simulink model "gaps_ut"  (Simulink 8.1)
settings: Solver=FixedStepDiscrete  StartTime=0.0  StopTime=10.0  FixedStep=0.005  RelTol=1e-3
libraries: siltestlib x11, gaps x1
settings Model: Creator=AT015126  LastModifiedBy=AT015555
settings DataIOCC: SignalLoggingSaveFormat=Dataset
settings OptimizationCC: ExpressionDepthLimit=128
settings DebuggingCC: FcnCallInpInsideContextMsg=EnableAllAsError
settings GRTTargetCC: CombineOutputUpdateFcns=on  GRTInterface=off

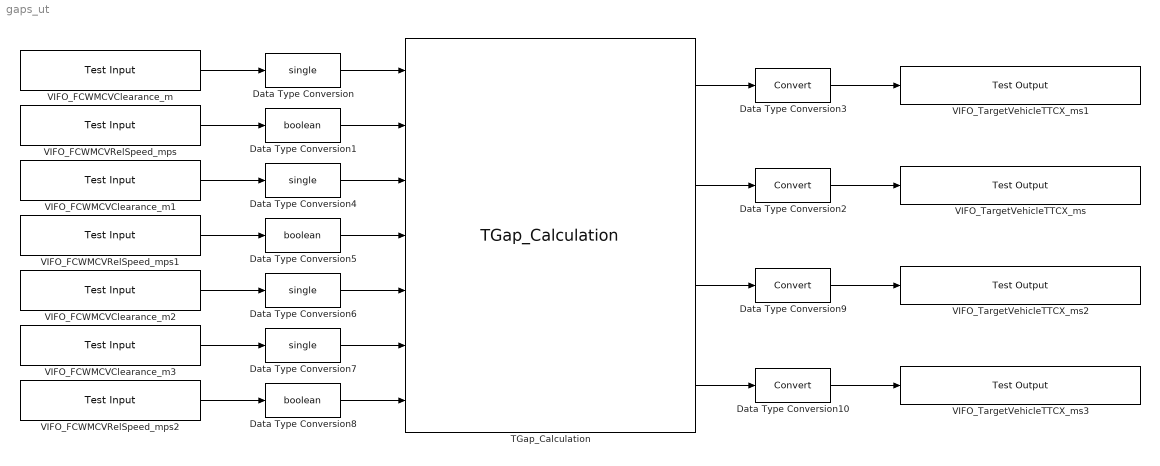
== system gaps_ut ==
  Data Type Conversion{,4,6..7} (4 alike) : DataTypeConversion  OutDataTypeStr=single
  Data Type Conversion1 : DataTypeConversion  OutDataTypeStr=boolean
  Data Type Conversion{2..3,9..10} (4 alike) : DataTypeConversion
  Data Type Conversion5 : DataTypeConversion  OutDataTypeStr=boolean
  Data Type Conversion8 : DataTypeConversion  OutDataTypeStr=boolean
  TGap_Calculation : gaps/TGap_Calculation
  VIFO_FCWMCVClearance_m : siltestlib/Test Input  varname=VIFO_AEBVehClearance_m  sampletime=0.005
  VIFO_FCWMCVClearance_m1 : siltestlib/Test Input  varname=VIFO_ACCMCVehXPosition_m  sampletime=0.005
  VIFO_FCWMCVClearance_m2 : siltestlib/Test Input  varname=VDINR_VehSpd_mps  sampletime=0.005
  VIFO_FCWMCVClearance_m3 : siltestlib/Test Input  varname=VIFO_FCWVehClearance_m  sampletime=0.005
  VIFO_FCWMCVRelSpeed_mps : siltestlib/Test Input  varname=VIFO_AEBTargetVehAssigned_flg  sampletime=0.005
  VIFO_FCWMCVRelSpeed_mps1 : siltestlib/Test Input  varname=VIFO_AEBTargetVehAssigned_flg  sampletime=0.005
  VIFO_FCWMCVRelSpeed_mps2 : siltestlib/Test Input  varname=VIFO_FCWTargetVehAssigned_flg  sampletime=0.005
  VIFO_TargetVehicleTTCX_ms : siltestlib/Test Output  varname=VIFO_ACCTGap_s  sampletime=-1
  VIFO_TargetVehicleTTCX_ms1 : siltestlib/Test Output  varname=VIFO_ACCVehClearance_m  sampletime=-1
  VIFO_TargetVehicleTTCX_ms2 : siltestlib/Test Output  varname=VIFO_AEBTGap_s  sampletime=-1
  VIFO_TargetVehicleTTCX_ms3 : siltestlib/Test Output  varname=VIFO_FCWTGap_s  sampletime=-1
  wires:
  VIFO_FCWMCVClearance_m/1 -> Data Type Conversion/1
  VIFO_FCWMCVRelSpeed_mps/1 -> Data Type Conversion1/1
  Data Type Conversion/1 -> TGap_Calculation/1
  Data Type Conversion1/1 -> TGap_Calculation/2
  Data Type Conversion2/1 -> VIFO_TargetVehicleTTCX_ms/1
  TGap_Calculation/2 -> Data Type Conversion2/1
  Data Type Conversion3/1 -> VIFO_TargetVehicleTTCX_ms1/1
  TGap_Calculation/1 -> Data Type Conversion3/1
  VIFO_FCWMCVClearance_m1/1 -> Data Type Conversion4/1
  Data Type Conversion4/1 -> TGap_Calculation/3
  VIFO_FCWMCVRelSpeed_mps1/1 -> Data Type Conversion5/1
  Data Type Conversion5/1 -> TGap_Calculation/4
  VIFO_FCWMCVClearance_m2/1 -> Data Type Conversion6/1
  Data Type Conversion6/1 -> TGap_Calculation/5
  VIFO_FCWMCVClearance_m3/1 -> Data Type Conversion7/1
  Data Type Conversion7/1 -> TGap_Calculation/6
  VIFO_FCWMCVRelSpeed_mps2/1 -> Data Type Conversion8/1
  Data Type Conversion8/1 -> TGap_Calculation/7
  Data Type Conversion9/1 -> VIFO_TargetVehicleTTCX_ms2/1
  TGap_Calculation/3 -> Data Type Conversion9/1
  Data Type Conversion10/1 -> VIFO_TargetVehicleTTCX_ms3/1
  TGap_Calculation/4 -> Data Type Conversion10/1
